simulink library "findClosestPathParameter_ul"  (R2020a)
settings: Solver=VariableStepAuto  StartTime=0.0  StopTime=10.0  RelTol=1e-3
settings Model: Creator=Ayaz  LastModifiedBy=Ayaz

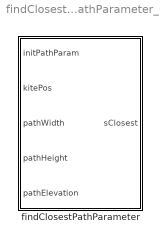
== system findClosestPathParameter_ul ==
  findClosestPathParameter : Subsystem

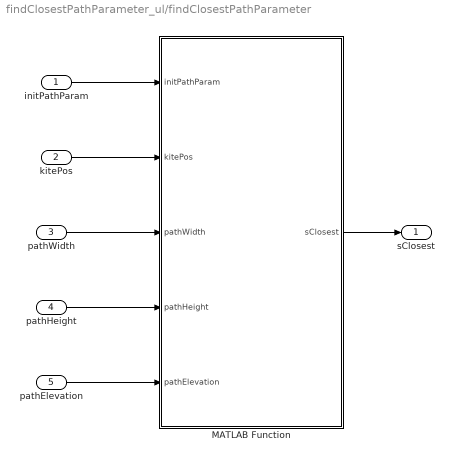
== system findClosestPathParameter_ul/findClosestPathParameter ==
  initPathParam : Inport
  kitePos : Inport  Port=2
  pathWidth : Inport  Port=3
  pathHeight : Inport  Port=4
  pathElevation : Inport  Port=5
  MATLAB Function : MATLAB Function  TreatAsAtomicUnit=on
  sClosest : Outport
  wires:
  initPathParam/1 -> MATLAB Function/1(initPathParam)
  kitePos/1 -> MATLAB Function/2(kitePos)
  pathElevation/1 -> MATLAB Function/5(pathElevation)
  pathHeight/1 -> MATLAB Function/4(pathHeight)
  pathWidth/1 -> MATLAB Function/3(pathWidth)
  MATLAB Function/1(sClosest) -> sClosest/1

== matlab function findClosestPathParameter_ul/findClosestPathParameter/MATLAB Function ==
  data: initPathParam input; kitePos input; sClosest output; pathWidth input; pathHeight input; pathElevation input
function sClosest = findClosestPathParameter(initPathParam,kitePos,...
    pathWidth,pathHeight,pathElevation)

sClosest = findClosestPathParameter(initPathParam,kitePos,...
    pathWidth,pathHeight,pathElevation);

end
